simulink model "SVPWM_Ti"  (R2021b)
settings: Solver=ode3  StartTime=0.0  StopTime=0.1  FixedStep=1e-5  RelTol=1e-3
libraries: dsparch4 x3, simulink x1, spsabctoAlphaBetaZeroLib x1, spspowerguiLib x1
settings Model: Creator=zyh  LastModifiedBy=zyh
settings SolverCC: AlgebraicLoopSolver=TrustRegion
settings DataIOCC: ReturnWorkspaceOutputs=off
settings DebuggingCC: MaskedZcDiagnostic=none  IgnoredZcDiagnostic=none  SFMachineParentedDataDiag=warning  ArithmeticOperatorsInVariantConditions=warning
settings SFSimCC: CustomCodeUndefinedFunction=UseInterfaceOnly

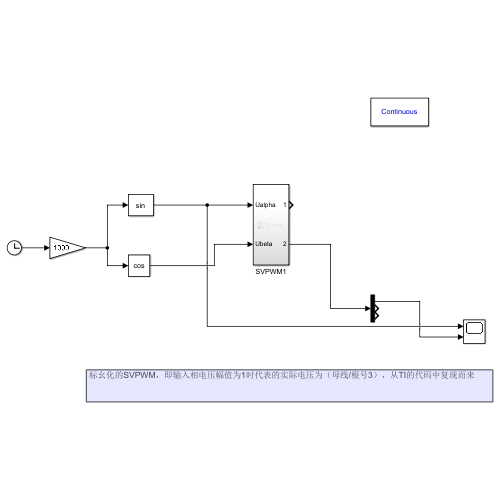
[thumbnail: Simulink's stored preview of the top-level diagram]
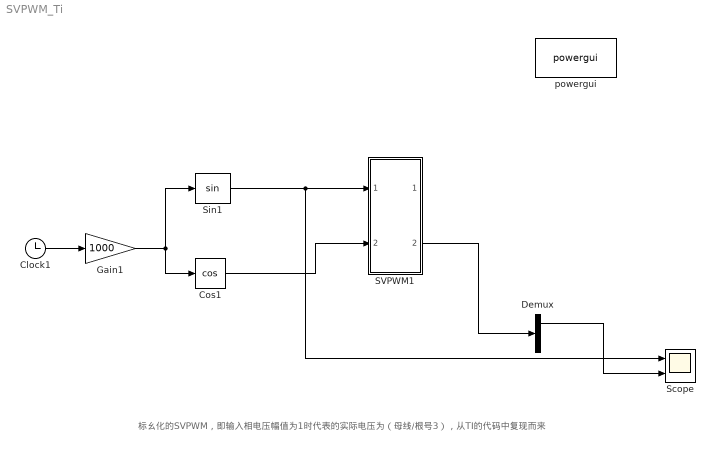
== system SVPWM_Ti ==
  note: 标幺化的SVPWM，即输入相电压幅值为1时代表的实际电压为（母线/根号3），从TI的代码中复现而来
  Clock1 : Clock
  Cos1 : Trigonometry  Operator=cos
  Demux : Demux  Outputs=3
  Gain1 : Gain  Gain=1000
  SVPWM1 : Subsystem
  Scope : Scope  NumInputPorts=2
  Sin1 : Trigonometry
  powergui : spspowerguiLib/powergui  Priority=1  SimulationMode=Continuous  SampleTime=1e-6  frequency=60  Iterations=50  frequencyindice=0  Pbase=100e6  ErrMax=1e-4  UnitsV=kV  UnitsW=MW  buscounter=0  FunctionMessages=off  echomessages=off  EnableUseOfTLC=off  CurrentSourceSwitches=off  DisableSnubberDevices=off  DisableRonSwitches=off  DisableVfSwitches=off  DisplayEquations=off  AutomaticDiscreteSolvers=off  SolverType=Tustin/Backward Euler (TBE)  Interpol=off  ExternalGateDelay=off  methode=off  Ts=100  x0status=blocks  SPID=on  SwTol=0  HookPort=off  NonlinearTolerance=1e-4  nMaxIteration=100  ContinueOnMaxIteration=off  RestoreLinks=warning  ResistiveCurrentMeasurement=off  Frange=[0:2:500]  Ylog=off  Xlog=on  ShowGrid=off  save=off  variable=ZData  structure=0  ZoomFFT=off  StartTime=0.0  cycles=1  DisplayStyle=1  fundamental=60  FreqAxis=off  MaxFrequency=1000  frequencyindicesteady=1  RmsSteady=1  display=off
  wires:
  Cos1/1 -> SVPWM1/2(Ubeta)
  Sin1/1 -> Scope/1, SVPWM1/1(Ualpha)
  Gain1/1 -> Sin1/1, Cos1/1
  Clock1/1 -> Gain1/1
  SVPWM1/2(Out2) -> Demux/1
  Demux/1 -> Scope/2

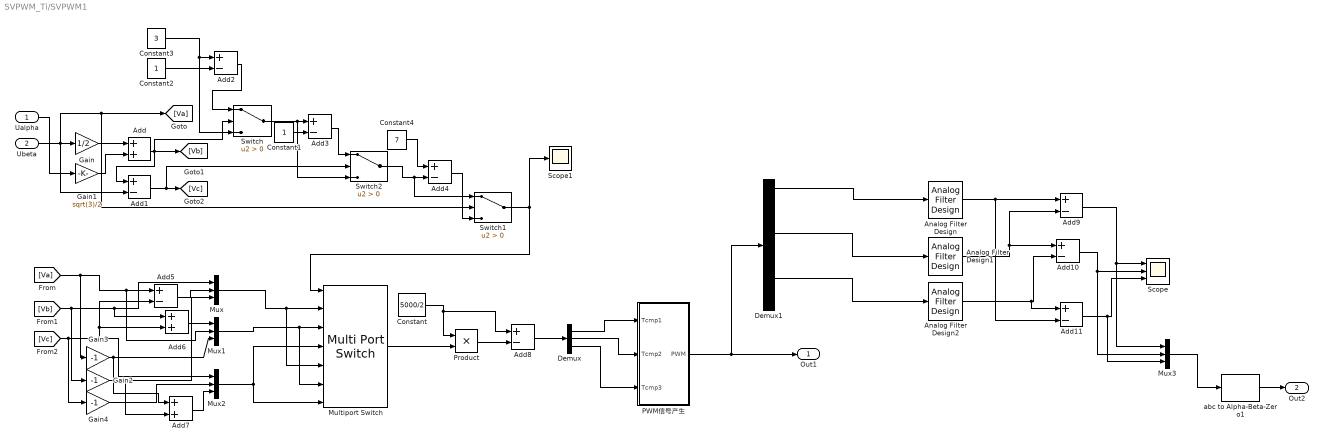
== system SVPWM_Ti/SVPWM1 ==
  Ualpha : Inport
  Ubeta : Inport  Port=2
  Add : Sum
  Add{1..5,8..11} (9 alike) : Sum  Inputs=+-
  Add6 : Sum
  Add7 : Sum
  Analog Filter Design : dsparch4/Analog Filter Design  method=Butterworth  filttype=Lowpass  N=2  Wlo=10000  Whi=80  Rp=2  Rs=40
  Analog Filter Design1 : dsparch4/Analog Filter Design  method=Butterworth  filttype=Lowpass  N=2  Wlo=10000  Whi=80  Rp=2  Rs=40
  Analog Filter Design2 : dsparch4/Analog Filter Design  method=Butterworth  filttype=Lowpass  N=2  Wlo=10000  Whi=80  Rp=2  Rs=40
  Constant : Constant  Value=5000/2
  Constant1 : Constant
  Constant2 : Constant
  Constant3 : Constant  Value=3
  Constant4 : Constant  Value=7
  Demux : Demux  Outputs=3
  Demux1 : Demux  Outputs=6
  Gain : Gain  Gain=1/2
  Gain1 : Gain  Gain=sqrt(3)/2
  Gain2 : Gain  Gain=-1
  Gain3 : Gain  Gain=-1
  Gain4 : Gain  Gain=-1
  Multiport Switch : MultiPortSwitch  Inputs=6  DiagnosticForDefault=None  OutDataTypeStr=double
  Mux{,1..3} (4 alike) : Mux  Inputs=3
  PWM信号产生 : Subsystem
  Product : Product
  Scope : Scope  NumInputPorts=3
  Scope1 : Scope
  Switch : Switch  Criteria=u2 > Threshold
  Switch1 : Switch  Criteria=u2 > Threshold
  Switch2 : Switch  Criteria=u2 > Threshold
  abc to Alpha-Beta-Zero1 : spsabctoAlphaBetaZeroLib/abc to Alpha-Beta-Zero
      settings: SourceProductBaseCode=PS
  Out1 : Outport  VectorParamsAs1DForOutWhenUnconnected=off
  Out2 : Outport  Port=2
  wires:
  PWM信号产生/1(PWM) -> Demux1/1, Out1/1
  Ualpha/1 -> Gain1/1
  Gain/1 -> Add/1
  Add/1 -> Switch/2, Add1/1, [Vb]
  Gain1/1 -> Add/2
  Ubeta/1 -> Add1/2, Gain/1, [Va], Switch1/2
  Add2/1 -> Switch/1
  Constant3/1 -> Switch/3, Add2/1
  Add1/1 -> Switch2/2, [Vc]
  Switch/1 -> Switch2/3, Add3/1
  Constant2/1 -> Add2/2
  Constant1/1 -> Add3/2
  Add3/1 -> Switch2/1
  Constant4/1 -> Add4/1
  Switch2/1 -> Switch1/1, Add4/2
  [Vb] -> Gain2/1, Add6/1, Mux/1
  [Va] -> Gain3/1, Mux1/2, Add5/1
  [Vc] -> Gain4/1, Mux2/1, Add6/2, Add5/2
  Add5/1 -> Mux/2
  Gain2/1 -> Add7/2, Mux/3
  Add6/1 -> Mux1/1
  Gain3/1 -> Add7/1, Mux1/3
  Gain4/1 -> Mux2/2
  Add7/1 -> Mux2/3
  Mux/1 -> Multiport Switch/5, Multiport Switch/2
  Mux1/1 -> Multiport Switch/6, Multiport Switch/3
  Mux2/1 -> Multiport Switch/4, Multiport Switch/7
  Constant/1 -> Add8/1, Product/1
  Multiport Switch/1 -> Product/2
  Add8/1 -> Demux/1
  Demux/1 -> PWM信号产生/1(Tcmp1)
  Demux/2 -> PWM信号产生/2(Tcmp2)
  Demux/3 -> PWM信号产生/3(Tcmp3)
  Switch1/1 -> Multiport Switch/1, Scope1/1
  Add4/1 -> Switch1/3
  Product/1 -> Add8/2
  Demux1/1 -> Analog Filter Design/1
  Demux1/3 -> Analog Filter Design1/1
  Demux1/5 -> Analog Filter Design2/1
  Analog Filter Design/1 -> Add11/2, Add9/1
  Analog Filter Design1/1 -> Add10/1, Add9/2
  Analog Filter Design2/1 -> Add11/1, Add10/2
  Add9/1 -> Mux3/1, Scope/1
  Add10/1 -> Mux3/2, Scope/2
  Add11/1 -> Mux3/3, Scope/3
  Mux3/1 -> abc to Alpha-Beta-Zero1/1
  abc to Alpha-Beta-Zero1/1 -> Out2/1

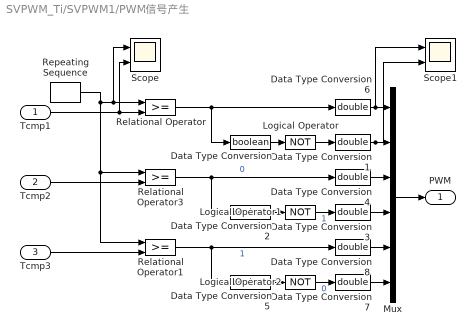
== system SVPWM_Ti/SVPWM1/PWM信号产生 ==
  Tcmp1 : Inport
  Tcmp2 : Inport  Port=2
  Tcmp3 : Inport  Port=3
  Data Type Conversion : DataTypeConversion  OutDataTypeStr=boolean
  Data Type Conversion{1,3..4,6..8} (6 alike) : DataTypeConversion  OutDataTypeStr=double
  Data Type Conversion2 : DataTypeConversion  OutDataTypeStr=boolean
  Data Type Conversion5 : DataTypeConversion  OutDataTypeStr=boolean
  Logical Operator : Logic  Operator=NOT  AllPortsSameDT=off  OutDataTypeStr=boolean
  Logical Operator1 : Logic  Operator=NOT  AllPortsSameDT=off  OutDataTypeStr=boolean
  Logical Operator2 : Logic  Operator=NOT  AllPortsSameDT=off  OutDataTypeStr=boolean
  Mux : Mux  Inputs=6
  Relational Operator : RelationalOperator  OutDataTypeStr=boolean  RndMeth=Nearest
  Relational Operator1 : RelationalOperator  OutDataTypeStr=boolean  RndMeth=Nearest
  Relational Operator3 : RelationalOperator  OutDataTypeStr=boolean  RndMeth=Nearest
  Repeating Sequence : simulink/Sources/Repeating Sequence  rep_seq_t=[0 1e-4 2e-4]  rep_seq_y=[0 5000 0]
  Scope : Scope  NumInputPorts=2
  Scope1 : Scope  NumInputPorts=2
  PWM : Outport  VectorParamsAs1DForOutWhenUnconnected=off
  wires:
  Data Type Conversion/1 -> Logical Operator/1
  Logical Operator/1 -> Data Type Conversion1/1
  Relational Operator/1 -> Data Type Conversion6/1, Data Type Conversion/1
  Logical Operator1/1 -> Data Type Conversion3/1  "1"
  Relational Operator3/1 -> Data Type Conversion4/1, Data Type Conversion2/1  "0"
  Data Type Conversion2/1 -> Logical Operator1/1
  Relational Operator1/1 -> Data Type Conversion8/1, Data Type Conversion5/1  "1"
  Data Type Conversion5/1 -> Logical Operator2/1
  Logical Operator2/1 -> Data Type Conversion7/1  "0"
  Repeating Sequence/1 -> Relational Operator1/1, Relational Operator3/1, Scope/1, Relational Operator/1
  Tcmp1/1 -> Scope/2, Relational Operator/2
  Tcmp2/1 -> Relational Operator3/2
  Tcmp3/1 -> Relational Operator1/2
  Data Type Conversion1/1 -> Scope1/2, Mux/2
  Data Type Conversion4/1 -> Mux/3
  Data Type Conversion3/1 -> Mux/4
  Data Type Conversion8/1 -> Mux/5
  Data Type Conversion7/1 -> Mux/6
  Mux/1 -> PWM/1
  Data Type Conversion6/1 -> Scope1/1, Mux/1
